simulink model "test_adcs"  (R2022b)
settings: Solver=VariableStepAuto  StartTime=0.0  StopTime=300  MaxStep=1e-1  RelTol=1e-3
settings Model: Creator=Jon  LastModifiedBy=Cal__
settings ModelReferenceCC: EnableRefExpFcnMdlSchedulingChecks=on

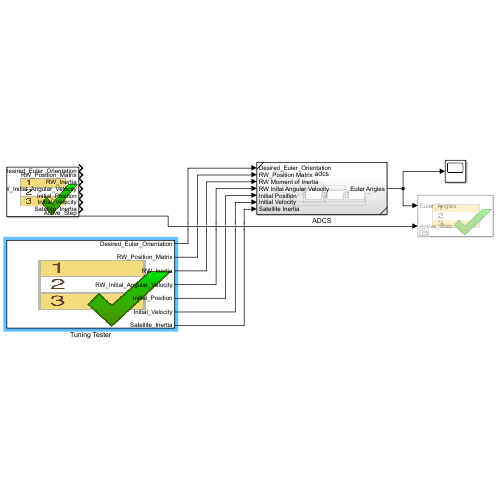
[thumbnail: Simulink's stored preview of the top-level diagram]
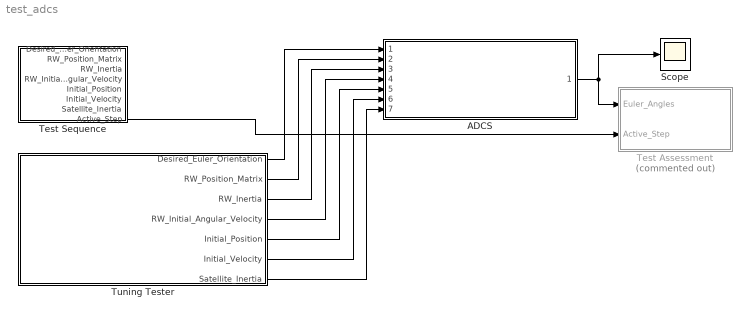
== system test_adcs ==
  ADCS : Subsystem  ReferencedSubsystem=adcs
  Scope : Scope
  Test Assessment : Test Sequence  Commented=on  TreatAsAtomicUnit=on
  Test Sequence : Test Sequence  TreatAsAtomicUnit=on
  Tuning Tester : Test Sequence  TreatAsAtomicUnit=on
  wires:
  Test Sequence/8(Active_Step) -> Test Assessment/2(Active_Step)
  ADCS/1 -> Scope/1, Test Assessment/1(Euler_Angles)
  Tuning Tester/1(Desired_Euler_Orientation) -> ADCS/1
  Tuning Tester/2(RW_Position_Matrix) -> ADCS/2
  Tuning Tester/3(RW_Inertia) -> ADCS/3
  Tuning Tester/4(RW_Initial_Angular_Velocity) -> ADCS/4
  Tuning Tester/5(Initial_Position) -> ADCS/5
  Tuning Tester/6(Initial_Velocity) -> ADCS/6
  Tuning Tester/7(Satellite_Inertia) -> ADCS/7

== stateflow chart test_adcs/Tuning Tester ==
  state Initialization
    RW_Inertia = 1e-7*92.5;
    RW_Position_Matrix = 1/sqrt(3)*[[1;1;-1],[1;-1;-1],[-1;-1;-1],[-1;1;-1]];
    Satellite_Inertia = 1e-9*[[20354701.41; 49833.89; 217681.32], [49833.89; 19938122.72; -75880.37], [217681.32; -75880.37; 5350609.8]];
    settings: description=Initialize test parameters
  state Test_Tuning
    RW_Initial_Angular_Velocity = [100; 0; 0; 0];
    Initial_Position = [0.5; 0.5; 0.5];
    Initial_Velocity = [0; 0; 0];
    Desired_Euler_Orientation = [0; 0; 0];
    settings: description=Test tuning
  (default) -> Initialization
  Initialization -> Test_Tuning : [
      | true
      | ]
  data: Desired_Euler_Orientation output; RW_Position_Matrix output; RW_Inertia output; RW_Initial_Angular_Velocity output; Initial_Position output; Initial_Velocity output; Satellite_Inertia output

== stateflow chart test_adcs/Test Assessment ==
  state Assessments
    state Verify_Zero
      verify(all(Euler_Angles == [0; 0; 0]))
    state Verify_Initial_Vel
      verify(all(Euler_Angles < 5e-3)) % 0.005 rad = 0.3 deg, requirement is 0.5 deg
    state Verify_Desired_Pos
      verify(all(Euler_Angles - [pi/2; pi/4; pi/6] < 5e-3))
    state Else
    (default) -> (junction 85)
    (junction 55) -> Verify_Zero [order 1] : [~in(Assessments.Verify_Zero)]
    (junction 85) -> (junction 55) [order 1] : [Active_Step == Active_Step_Enum.Test_Zero
        | ]
    (junction 55) -> (junction 58) [order 2]
    Assessments -> (junction 85)
    (junction 85) -> (junction 76) [order 2]
    (junction 76) -> (junction 77) [order 1] : [t > 60 && Active_Step == Active_Step_Enum.Test_Initial_Vel
        | ]
    (junction 77) -> Verify_Initial_Vel [order 1] : [~in(Assessments.Verify_Initial_Vel)]
    (junction 76) -> (junction 105) [order 2]
    (junction 77) -> (junction 80) [order 2]
    (junction 105) -> (junction 106) [order 1] : [t > 210 && Active_Step == Active_Step_Enum.Test_Desired_Pos
        | ]
    (junction 106) -> Verify_Desired_Pos [order 1] : [~in(Assessments.Verify_Desired_Pos)]
    (junction 105) -> (junction 96) [order 2]
    (junction 106) -> (junction 109) [order 2]
    (junction 96) -> (junction 97)
    (junction 97) -> Else [order 1] : [~in(Assessments.Else)]
    (junction 97) -> (junction 100) [order 2]
  (default) -> Assessments
  data: Euler_Angles input; Active_Step input

== stateflow chart test_adcs/Test Sequence ==
  state Initialization
    RW_Inertia = 1e-7*92.5;
    RW_Position_Matrix = 1/sqrt(3)*[[1;1;-1],[1;-1;-1],[-1;-1;-1],[-1;1;-1]];
    Satellite_Inertia = 1e-9*[[20354701.41; 49833.89; 217681.32], [49833.89; 19938122.72; -75880.37], [217681.32; -75880.37; 5350609.8]];
    settings: description=Initialize test parameters
  state Test_Zero
    Desired_Euler_Orientation = [0; 0; 0];
    Initial_Position = [0; 0; 0];
    RW_Initial_Angular_Velocity = [0; 0; 0; 0];
    Initial_Position = [0; 0; 0];
    Initial_Velocity = [0; 0; 0];
    settings: description=Test no movement
  state Test_Initial_Vel
    Initial_Velocity = [0; pi/4; 0];
    settings: description=Test cancelling initial velocity
  state Test_Desired_Pos
    Desired_Euler_Orientation = [pi/2; pi/4; pi/6];
    settings: description=Test giving desired orientation
  (default) -> Initialization
  Initialization -> Test_Zero : [
      | true
      | ]
  Test_Zero -> Test_Initial_Vel : [
      | after(1, sec)
      | ]
  Test_Initial_Vel -> Test_Desired_Pos : [
      | after(90, sec)
      | ]
  data: Desired_Euler_Orientation output; RW_Position_Matrix output; RW_Inertia output; RW_Initial_Angular_Velocity output; Initial_Position output; Initial_Velocity output; Satellite_Inertia output; Active_Step output Enum: Active_Step_Enum
